simulink model "es2_catena_chiusa_2"  (R2014a)
settings: Solver=ode45  StartTime=0.0  StopTime=40.0  RelTol=1e-3
values from neighbouring files (symbols this model uses):
  F1 = (Ka * Km) / (s^2 * J * La + s * (beta * La + J * Ra) + beta * Ra + Km^2)    [es2.m]
  F2 = -(s * La + Ra) / (s^2 * J * La + s * (beta * La + J * Ra) + beta * Ra + Km^2)    [es2.m]
  Kc = 1    [es2.m]
  s = tf('s')    [es2.m]
libraries: cstblocks x2
settings Model: Creator=HP  LastModifiedBy=HP

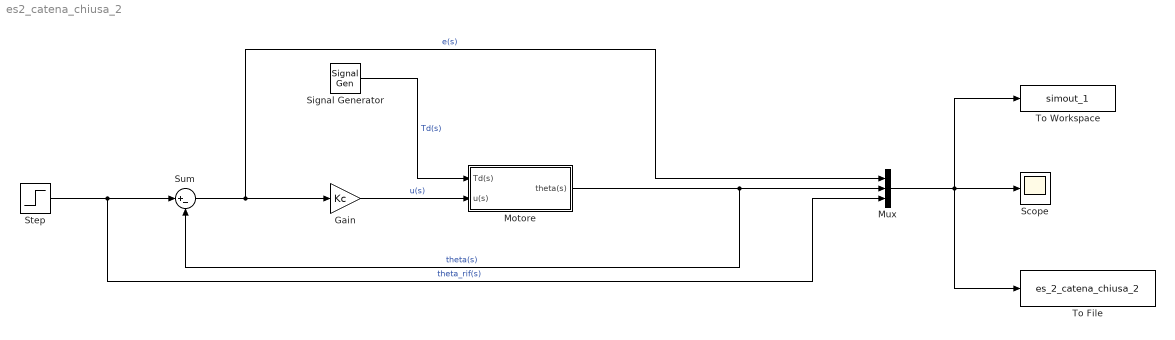
== system es2_catena_chiusa_2 ==
  Gain : Gain  Gain=Kc
  Motore : Subsystem  TreatAsAtomicUnit=on
  Mux : Mux  Inputs=3
  Scope : Scope
      settings: MaxDataPoints=100000
  Signal Generator : SignalGenerator  WaveForm=square  Amplitude=0.05  Frequency=0.1
  Step : Step  Time=0  SampleTime=0
  Sum : Sum  Inputs=|+-
  To File : ToFile  Filename=es_2_catena_chiusa_2  MatrixName=output_2  SaveFormat=Timeseries
  To Workspace : ToWorkspace  VariableName=simout_1  SaveFormat=Timeseries  SampleTime=-1
  wires:
  Gain/1 -> Motore/2(u(s))  "u(s)"
  Step/1 -> Mux/3, Sum/1  "theta_rif(s)"
  Sum/1 -> Mux/1, Gain/1  "e(s)"
  Signal Generator/1 -> Motore/1(Td(s))  "Td(s)"
  Motore/1(theta(s)) -> Sum/2, Mux/2  "theta(s)"
  Mux/1 -> To Workspace/1, To File/1, Scope/1

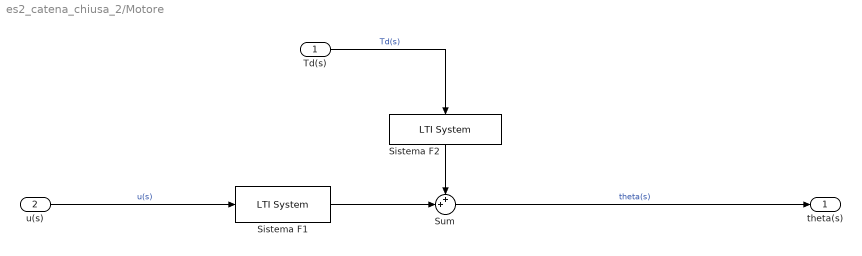
== system es2_catena_chiusa_2/Motore ==
  Td(s) : Inport
  u(s) : Inport  Port=2
  Sistema F1 : cstblocks/LTI System  sys=F1/s  IC=[]
  Sistema F2 : cstblocks/LTI System  sys=F2/s  IC=[]
  Sum : Sum  Inputs=++|
  theta(s) : Outport
  wires:
  u(s)/1 -> Sistema F1/1  "u(s)"
  Sistema F1/1 -> Sum/2
  Sistema F2/1 -> Sum/1
  Td(s)/1 -> Sistema F2/1  "Td(s)"
  Sum/1 -> theta(s)/1  "theta(s)"
